simulink library "mmuct_lib"  (R2025a)
settings: Solver=VariableStepAuto  StartTime=0.0  StopTime=10.0  RelTol=1e-3
undefined symbols (not defined in the file): fractalcoef, simstruct, struct2bus
libraries: $bdroot x2, dhaouadi2013_lib x2, mspsensorlib x1
settings Model: Creator=nicolls  LastModifiedBy=MTMTAD006

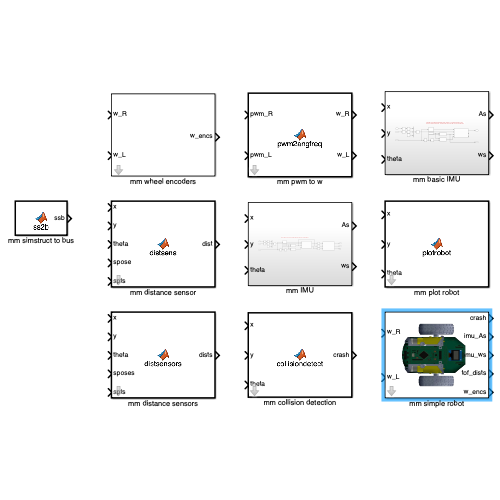
[thumbnail: Simulink's stored preview of the top-level diagram]
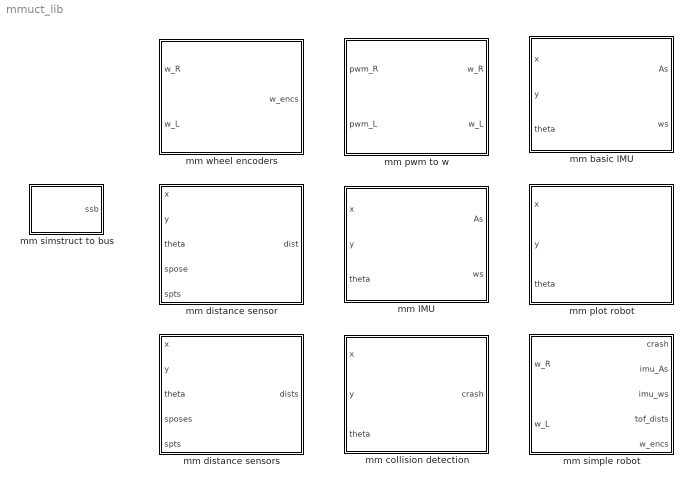
== system mmuct_lib ==
  mm IMU : Subsystem
  mm basic IMU : Subsystem
  mm collision detection : MATLAB Function  InitFcn=struct2bus(simstruct,'ssbus');  TreatAsAtomicUnit=on  mask(MM Collision Detection){simstruct=simstruct}
      mask prompts: simstruct "Simulation structure variable"
      mask help:
      | Detect crash for UCT micromouse at specified pose (x, y, theta) on map.
      |
      | This function uses a simulation structure variable that must include fields "mapim", "mapres", and "robot_rad".
  mm distance sensor : MATLAB Function  InitFcn=struct2bus(simstruct,'ssbus');  TreatAsAtomicUnit=on  mask(MM Distance Sensor){simstruct=simstruct, debug=0}
      mask prompts: simstruct "Simulation structure variable"; debug "Display debugging output"
      mask help:
      | Generate measurement for distance sensor mounted on UCT micro-mouse.  The robot is assumed to be located at pose (x, y, theta) in a map specified by the simulation structure variable.  The sensor is at pose "spose" (x, y, theta) relative to the robot coordinate frame, where the robot kinematic center is at the origin and the forward direction is along the x axis.  The function works by evaluating the map at sensor locations specified by spts, and returns the point corresponding to the closest collision.
      |
      | This function uses a simulation structure variable that must include fields "mapim" and "mapres".
  mm distance sensors : MATLAB Function  InitFcn=struct2bus(simstruct,'ssbus');  TreatAsAtomicUnit=on  mask(MM Distance Sensor){simstruct=simstruct, debug=1}
      mask prompts: simstruct "Simulation structure variable"; debug "Display debugging output"
      mask help:
      | Generate measurement for distance sensor mounted on UCT micro-mouse.  The robot is assumed to be located at pose (x, y, theta) in a map specified by the simulation structure variable.  The sensor is at pose "spose" (x, y, theta) relative to the robot coordinate frame, where the robot kinematic center is at the origin and the forward direction is along the x axis.  The function works by evaluating the map at sensor locations specified by spts, and returns the point corresponding to the closest collision.
      |
      | This function uses a simulation structure variable that must include fields "mapim" and "mapres".
  mm plot robot : MATLAB Function  InitFcn=|  TreatAsAtomicUnit=on  mask(MM Plot Robot){x0=0.1, y0=0.1, theta0=0, simstruct=simstruct}
      | simstruct_var = get_param(gcb,'simstruct'); 
      | existsinbase = evalin('base', ['exist(''' simstruct_var ''',''var'')']); 
      | 
      | ss = [];
      | if existsinbase 
      |   %disp(['initFcn: loading simulation structure ' simstruct_var]); 
      |   ss = evalin('base',simstruct_var); 
      | end
      | struct2bus(ss,'ssbus');  % generate bus definition
      mask prompts: x0 "x0 (m)"; y0 "y0 (m)"; theta0 "theta0 (rad)"; simstruct "Simulation structure variable"
      mask help:
      | Plot UCT micromouse at specified pose (x, y, theta) on map.
      |
      | This function uses a simulation structure variable that must include fields "mapim", "mapres", "robot_img", "robot_imgalpha", and "robot_imgxyd".  It also opens a figure and leaves a handle "UCTMMRobotSimulatorHandle" in the base workspace.
      mask init:
      | FigureName = 'UCT MM Robot Simulator';
      |   FigureTag = 'UCTMMRobotSimulator';
      | 
      |   h = findobj('Name',FigureName);
      |   if ~isempty(h)
      |     close (h); 
      |   end
      | 
      |   % Figure setup
      |   existingFigures = findobj('type','figure','tag',FigureTag);
      |   if ~isempty(existingFigures)
      |     figure(existingFigures(1)); % bring figure to the front
      |     error('There is already an existing figure window for RobotSimulator.');
      |   end
      |   fh = figure('Name',FigureName,'tag',FigureTag);
      |   ax = axes('parent',fh);
      | 
      |   % % Mask parameters
      |   % x0 = str2double(get_param(gcb,'x0'));
      |   % y0 = str2double(get_param(gcb,'y0'));
      |   % theta0 = str2double(get_param(gcb,'theta0'));
      |   % 
      |   % % Determine if simstruct is available
      |   % simstruct = [];
      |   % simstruct_var = get_param(gcb,'simstruct');
      |   % existsinbase = evalin('base', ['exist(''' simstruct_var ''',''var'')']);
      |   % if existsinbase
      |   %   simstruct = evalin('base',simstruct_var);
      |   % end
      | 
      |   % Display map
      |   if isfield(simstruct,'mapim') && isfield(simstruct,'mapres')
      |     map = binaryOccupancyMap(simstruct.mapim,simstruct.mapres);
      |     show(map,'Parent',ax); 
      |   else
      |     axis([-2 2 -2 2]);
      |   end
      | 
      |   % Display robot
      |   if isfield(simstruct,'robot_img') && isfield(simstruct,'robot_imgalpha') && isfield(simstruct,'robot_imgxyd')
      |     % Get robot
      |     robot_img = simstruct.robot_img;
      |     robot_imgalpha = simstruct.robot_imgalpha;
      |     robot_imgxyd = simstruct.robot_imgxyd;
      | 
      |     % Display robot
      |     robot_imgr = imrotate(robot_img,-theta0*180/pi,'crop');
      |     robot_imgalphar = imrotate(robot_imgalpha,-theta0*180/pi,'crop');
      |     hold on;
      |     ih = image(x0+robot_imgxyd,y0+robot_imgxyd,robot_imgr);
      |     set(ih,'AlphaData',robot_imgalphar);
      |     hold off;
      |   else
      |     hold on;  sh = scatter(x0,y0,'ro');  hold off;
      |     llen = 0.25;
      |     hold on;  lh = line([x0; x0+llen*cos(theta0)],[y0;y0+llen*sin(theta0)]);  hold off;
      |     ih = [sh lh];
      |   end
      | 
      |   % Store handles 
      |   set(fh,'UserData',ih);
      |   assignin('base','UCTMMRobotSimulatorHandle',fh);
  mm pwm to w : MATLAB Function  TreatAsAtomicUnit=on  mask{deadb=30, maxw=2*pi}
      mask prompts: deadb "Dead band (%)"; maxw "Max. angular velocity (rad/s)"
  mm simple robot : Subsystem  mask{simstruct=simstruct, x0=0.1, y0=0.1, theta0=0}
      mask prompts: simstruct "Simulation structure variable"; x0 "x0 (m)"; y0 "y0 (m)"; theta0 "theta0 (rad)"
      mask DialogControl Container3 Prompt: Initial pose
      mask Display: image('uctmm_image.png');
  mm simstruct to bus : MATLAB Function  InitFcn=struct2bus(simstruct,'ssbus')  TreatAsAtomicUnit=on
  mm wheel encoders : Subsystem  mask{ticsperrev=12}
      mask prompts: ticsperrev "Tics/rev"

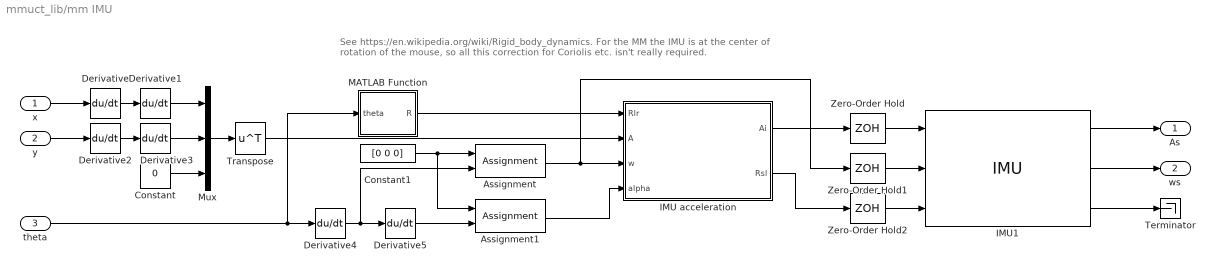
== system mmuct_lib/mm IMU ==
  note: See https://en.wikipedia.org/wiki/Rigid_body_dynamics. For the MM the IMU is at the center of rotation of the mouse, so all this correction for Coriolis etc. isn't really required.
  x : Inport
  y : Inport  Port=2
  theta : Inport  Port=3
  Assignment : Assignment  DiagnosticForDimensions=Warning  IndexOptions=Index vector (dialog)  Indices=3  OutputSizes=1
  Assignment1 : Assignment  DiagnosticForDimensions=Warning  IndexOptions=Index vector (dialog)  Indices=3  OutputSizes=1
  Constant : Constant  Value=0
  Constant1 : Constant  Value=[0 0 0]  VectorParams1D=off
  Derivative{,1..5} (6 alike) : Derivative
  IMU acceleration : MATLAB Function  TreatAsAtomicUnit=on
  IMU1 : mspsensorlib/IMU  DispRefFrame=ENU  TemperaturePort=off  Temperature=25  MagneticFieldPort=off  MagneticFieldNED=[ 27.5550, -2.4169, -16.0849 ]  MagneticFieldENU=[ -2.4169, 27.5550, 16.0849 ]  SeedDouble=67  SimulateUsing=Interpreted execution  AccelParamsMeasurementRange=Inf  AccelParamsResolution=0  AccelParamsConstantBias=[ 0, 0, 0 ]  AccelParamsAxesMisalignment=[ 100, 0, 0; 0, 100, 0; 0, 0, 100 ]  AccelParamsNoiseDensity=[ 0, 0, 0 ]  AccelParamsBiasInstability=[ 0, 0, 0 ]  AccelParamsBiasInstabilityNumerator=fractalcoef().Numerator  AccelParamsBiasInstabilityDenominator=fractalcoef().Denominator  AccelParamsRandomWalk=[ 0, 0, 0 ]  AccelParamsNoiseType=double-sided  AccelParamsTemperatureBias=[ 0, 0, 0 ]  AccelParamsTemperatureScaleFactor=[ 0, 0, 0 ]  GyroParamsMeasurementRange=Inf  GyroParamsResolution=0  GyroParamsConstantBias=[ 0, 0, 0 ]  GyroParamsAxesMisalignment=[ 100, 0, 0; 0, 100, 0; 0, 0, 100 ]  GyroParamsAccelerationBias=[ 0, 0, 0 ]  GyroParamsNoiseDensity=[ 0, 0, 0 ]  GyroParamsBiasInstability=[ 0, 0, 0 ]  GyroParamsBiasInstabilityNumerator=fractalcoef().Numerator  GyroParamsBiasInstabilityDenominator=fractalcoef().Denominator  GyroParamsRandomWalk=[ 0, 0, 0 ]  GyroParamsNoiseType=double-sided  GyroParamsTemperatureBias=[ 0, 0, 0 ]  GyroParamsTemperatureScaleFactor=[ 0, 0, 0 ]  MagParamsMeasurementRange=Inf  MagParamsResolution=0  MagParamsConstantBias=[ 0, 0, 0 ]  MagParamsAxesMisalignment=[ 100, 0, 0; 0, 100, 0; 0, 0, 100 ]  MagParamsNoiseDensity=[ 0, 0, 0 ]  MagParamsBiasInstability=[ 0, 0, 0 ]  MagParamsBiasInstabilityNumerator=fractalcoef().Numerator  MagParamsBiasInstabilityDenominator=fractalcoef().Denominator  MagParamsRandomWalk=[ 0, 0, 0 ]  MagParamsNoiseType=double-sided  MagParamsTemperatureBias=[ 0, 0, 0 ]  MagParamsTemperatureScaleFactor=[ 0, 0, 0 ]
  MATLAB Function : MATLAB Function  TreatAsAtomicUnit=on
  Mux : Mux  Inputs=3
  Terminator : Terminator
  Transpose : Math  Operator=transpose
  Zero-Order Hold : ZeroOrderHold  SampleTime=0.02
  Zero-Order Hold1 : ZeroOrderHold  SampleTime=0.02
  Zero-Order Hold2 : ZeroOrderHold  SampleTime=0.02
  As : Outport
  ws : Outport  Port=2
  wires:
  IMU acceleration/2(Rsl) -> Zero-Order Hold2/1
  Mux/1 -> Transpose/1
  IMU acceleration/1(Ai) -> Zero-Order Hold/1
  Zero-Order Hold/1 -> IMU1/1
  Zero-Order Hold1/1 -> IMU1/2
  IMU1/1 -> As/1
  Zero-Order Hold2/1 -> IMU1/3
  x/1 -> Derivative/1
  Derivative/1 -> Derivative1/1
  Derivative2/1 -> Derivative3/1
  y/1 -> Derivative2/1
  Derivative1/1 -> Mux/1
  Derivative3/1 -> Mux/2
  Constant/1 -> Mux/3
  IMU1/2 -> ws/1
  theta/1 -> MATLAB Function/1(theta), Derivative4/1
  MATLAB Function/1(R) -> IMU acceleration/1(Rlr)
  Constant1/1 -> Assignment1/1, Assignment/1
  Derivative4/1 -> Assignment/2, Derivative5/1
  Assignment/1 -> Zero-Order Hold1/1, IMU acceleration/3(w)
  Derivative5/1 -> Assignment1/2
  Assignment1/1 -> IMU acceleration/4(alpha)
  Transpose/1 -> IMU acceleration/2(A)
  IMU1/3 -> Terminator/1

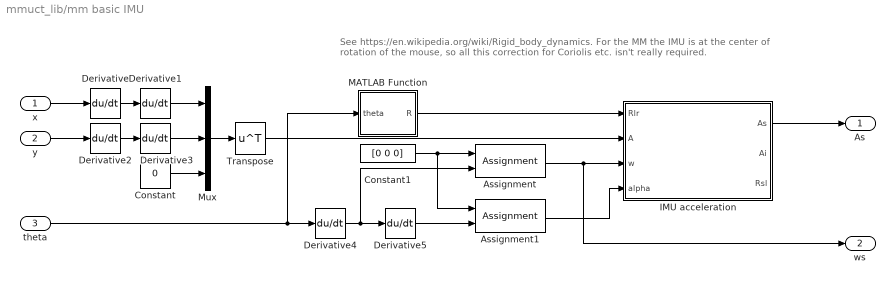
== system mmuct_lib/mm basic IMU ==
  note: See https://en.wikipedia.org/wiki/Rigid_body_dynamics. For the MM the IMU is at the center of rotation of the mouse, so all this correction for Coriolis etc. isn't really required.
  x : Inport
  y : Inport  Port=2
  theta : Inport  Port=3
  Assignment : Assignment  DiagnosticForDimensions=Warning  IndexOptions=Index vector (dialog)  Indices=3  OutputSizes=1
  Assignment1 : Assignment  DiagnosticForDimensions=Warning  IndexOptions=Index vector (dialog)  Indices=3  OutputSizes=1
  Constant : Constant  Value=0
  Constant1 : Constant  Value=[0 0 0]  VectorParams1D=off
  Derivative{,1..5} (6 alike) : Derivative
  IMU acceleration : MATLAB Function  TreatAsAtomicUnit=on
  MATLAB Function : MATLAB Function  TreatAsAtomicUnit=on
  Mux : Mux  Inputs=3
  Transpose : Math  Operator=transpose
  As : Outport
  ws : Outport  Port=2
  wires:
  Assignment1/1 -> IMU acceleration/4(alpha)
  Derivative5/1 -> Assignment1/2
  Assignment/1 -> ws/1, IMU acceleration/3(w)
  Derivative4/1 -> Derivative5/1, Assignment/2
  Constant1/1 -> Assignment/1, Assignment1/1
  MATLAB Function/1(R) -> IMU acceleration/1(Rlr)
  theta/1 -> Derivative4/1, MATLAB Function/1(theta)
  Constant/1 -> Mux/3
  Derivative3/1 -> Mux/2
  Derivative1/1 -> Mux/1
  y/1 -> Derivative2/1
  Derivative2/1 -> Derivative3/1
  Derivative/1 -> Derivative1/1
  x/1 -> Derivative/1
  Mux/1 -> Transpose/1
  Transpose/1 -> IMU acceleration/2(A)
  IMU acceleration/1(As) -> As/1

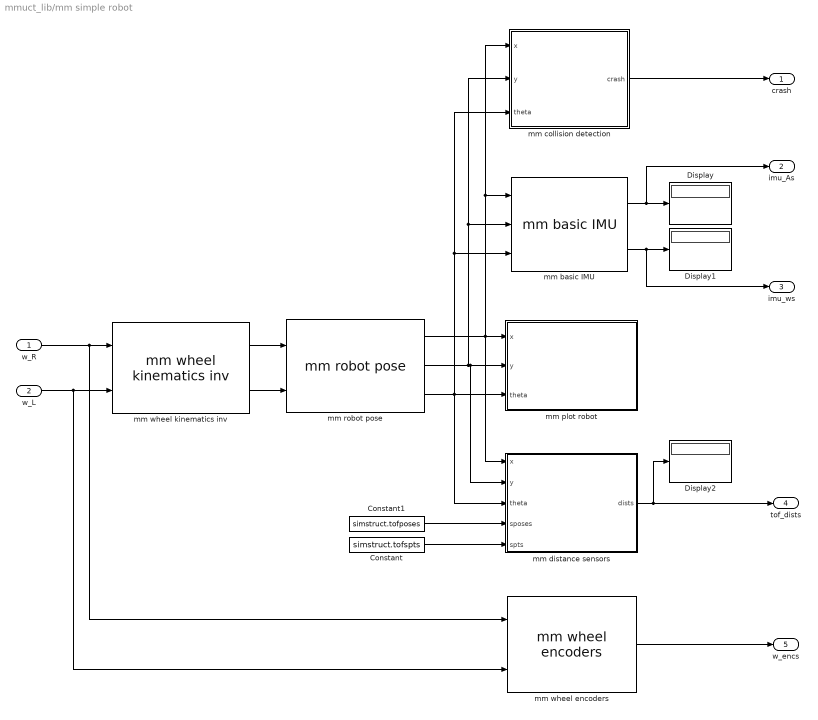
== system mmuct_lib/mm simple robot ==
  w_R : Inport
  w_L : Inport  Port=2
  Constant : Constant  Value=simstruct.tofspts
  Constant1 : Constant  Value=simstruct.tofposes
  Display : Display
  Display1 : Display
  Display2 : Display
  mm basic IMU : $bdroot/mm basic IMU  SystemSampleTime=-1  VariantActivationTime=update diagram  EmptyChoice=off  PassThrough=off  PassThroughVariantControl=(default)  EmptyChoiceVariantControl=(default)  AllowFlexibleInterface=on  Latency=0  AutoFrameSizeCalculation=off
  mm collision detection : MATLAB Function  InitFcn=struct2bus(simstruct,'ssbus');  TreatAsAtomicUnit=on  mask(MM Collision Detection){simstruct=simstruct}
      mask prompts: simstruct "Simulation structure variable"
      mask help:
      | Detect crash for UCT micromouse at specified pose (x, y, theta) on map.
      |
      | This function uses a simulation structure variable that must include fields "mapim", "mapres", and "robot_rad".
  mm distance sensors : MATLAB Function  InitFcn=struct2bus(simstruct,'ssbus');  TreatAsAtomicUnit=on  mask(MM Distance Sensor){simstruct=simstruct, debug=0}
      mask prompts: simstruct "Simulation structure variable"; debug "Display debugging output"
      mask help:
      | Generate measurement for distance sensor mounted on UCT micro-mouse.  The robot is assumed to be located at pose (x, y, theta) in a map specified by the simulation structure variable.  The sensor is at pose "spose" (x, y, theta) relative to the robot coordinate frame, where the robot kinematic center is at the origin and the forward direction is along the x axis.  The function works by evaluating the map at sensor locations specified by spts, and returns the point corresponding to the closest collision.
      |
      | This function uses a simulation structure variable that must include fields "mapim" and "mapres".
  mm plot robot : MATLAB Function  InitFcn=|  TreatAsAtomicUnit=on  mask(MM Plot Robot){x0=x0, y0=y0, theta0=theta0, simstruct=simstruct}
      | simstruct_var = get_param(gcb,'simstruct'); 
      | existsinbase = evalin('base', ['exist(''' simstruct_var ''',''var'')']); 
      | 
      | ss = [];
      | if existsinbase 
      |   %disp(['initFcn: loading simulation structure ' simstruct_var]); 
      |   ss = evalin('base',simstruct_var); 
      | end
      | struct2bus(ss,'ssbus');  % generate bus definition
      mask prompts: x0 "x0 (m)"; y0 "y0 (m)"; theta0 "theta0 (rad)"; simstruct "Simulation structure variable"
      mask help:
      | Plot UCT micromouse at specified pose (x, y, theta) on map.
      |
      | This function uses a simulation structure variable that must include fields "mapim", "mapres", "robot_img", "robot_imgalpha", and "robot_imgxyd".  It also opens a figure and leaves a handle "UCTMMRobotSimulatorHandle" in the base workspace.
      mask init: same as mmuct_lib/mm plot robot
  mm robot pose : dhaouadi2013_lib/mm robot pose  x0=x0  y0=y0  theta0=0
  mm wheel encoders : $bdroot/mm wheel encoders  ticsperrev=8
  mm wheel kinematics inv : dhaouadi2013_lib/mm wheel kinematics inv  L=simstruct.L  R=simstruct.R
  crash : Outport
  imu_As : Outport  Port=2
  imu_ws : Outport  Port=3
  tof_dists : Outport  Port=4
  w_encs : Outport  Port=5
  wires:
  mm wheel encoders/1 -> w_encs/1
  mm distance sensors/1(dists) -> tof_dists/1, Display2/1
  Constant/1 -> mm distance sensors/5(spts)
  Constant1/1 -> mm distance sensors/4(sposes)
  mm wheel kinematics inv/2 -> mm robot pose/2
  mm robot pose/2 -> mm plot robot/2(y), mm distance sensors/2(y), mm collision detection/2(y), mm basic IMU/2
  mm basic IMU/2 -> imu_ws/1, Display1/1
  mm basic IMU/1 -> Display/1, imu_As/1
  mm wheel kinematics inv/1 -> mm robot pose/1
  mm robot pose/1 -> mm plot robot/1(x), mm basic IMU/1, mm collision detection/1(x), mm distance sensors/1(x)
  mm robot pose/3 -> mm plot robot/3(theta), mm collision detection/3(theta), mm basic IMU/3, mm distance sensors/3(theta)
  mm collision detection/1(crash) -> crash/1
  w_L/1 -> mm wheel kinematics inv/2, mm wheel encoders/2
  w_R/1 -> mm wheel kinematics inv/1, mm wheel encoders/1

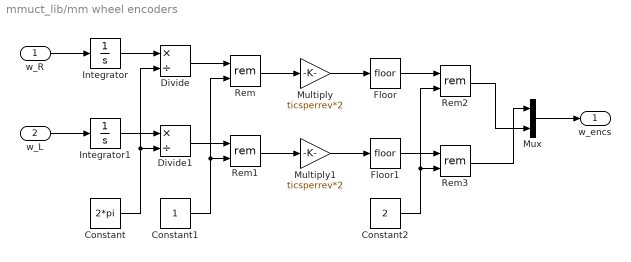
== system mmuct_lib/mm wheel encoders ==
  w_R : Inport
  w_L : Inport  Port=2
  Constant : Constant  Value=2*pi
  Constant1 : Constant
  Constant2 : Constant  Value=2
  Divide : Product  Inputs=*/
  Divide1 : Product  Inputs=*/
  Floor : Rounding
  Floor1 : Rounding
  Integrator : Integrator
  Integrator1 : Integrator
  Multiply : Gain  Gain=ticsperrev*2
  Multiply1 : Gain  Gain=ticsperrev*2
  Mux : Mux  Inputs=2
  Rem{,1..3} (4 alike) : Math  Operator=rem
  w_encs : Outport
  wires:
  Mux/1 -> w_encs/1
  Rem3/1 -> Mux/1
  Rem2/1 -> Mux/2
  Constant2/1 -> Rem2/2, Rem3/2
  Floor/1 -> Rem2/1
  Floor1/1 -> Rem3/1
  Multiply1/1 -> Floor1/1
  Multiply/1 -> Floor/1
  Rem/1 -> Multiply/1
  Rem1/1 -> Multiply1/1
  Constant1/1 -> Rem/2, Rem1/2
  Divide1/1 -> Rem1/1
  Divide/1 -> Rem/1
  Constant/1 -> Divide/2, Divide1/2
  Integrator1/1 -> Divide1/1
  Integrator/1 -> Divide/1
  w_L/1 -> Integrator1/1
  w_R/1 -> Integrator/1

== matlab function mmuct_lib/mm distance sensors ==
  data: x input; y input; theta input; dists output; sposes input; spts input; simstruct parameter; debug parameter
function dists = distsensors(x,y,theta,sposes,spts,simstruct,debug)
%DISTSENS  Simulate output of time-of-flight distance sensor
%   dists = distsens(x,y,theta,sposes,spts,simstruct,debug) takes a
%   robot pose in the world (x, y, theta), a sensor pose in the robot frame
%   (spos), and a set of sensor points to be checked in the sensor frame,
%   and finds the distance from the sensor to the nearest sensor point that
%   collides with an occupied cell on a map. 
%
%   Parameters:
%     x, y, theta - robot pose in world
%     sposes - sensor poses in robot frame (one row [x y theta] for each
%              sensor).  It is assumed that the robot is centered at the
%              origin and is pointing forwards along the x axis 
%     spts - set of points in sensor frame for which to detect collisions.
%            Must be increasing and should be spaced closely enough for
%            collisions to be detected
%     simstruct - simulation structure assumed to have field mapim for map
%                 occupancy image (zero for cell unoccupied), at a map
%                 resolution mapres (pixels per meter)
%     debug - display interesting plot
%
%   Fred Nicolls, July 2025

coder.extrinsic('get_param','set_param');

rpose = [x y theta]';
if numel(rpose)~=3, error('Invalid dimension'); end
if size(sposes,2)~=3, error('Invalid dimension'); end
if any(diff(spts)<0), error('Sensor points must be increasing'); end
if nargin<7, debug=0; end
numsens = size(sposes,1);

% Transpose inputs if required
if size(rpose,1)==1, rpose = rpose'; end
if size(spts,1)==1, sptsr = spts;  else sptsr = spts'; end

% Points in sensor frame lying on x-axis
xs = [sptsr; zeros(size(sptsr))];

% Robot to world coordinate transformation
thetar = rpose(3);  xyr = rpose(1:2);
Rwr = [cos(thetar) -sin(thetar) xyr(1); sin(thetar) cos(thetar) xyr(2); 0 0 1];

% Collect sensor information in cells
Rrsc = cell(numsens,1);
xwsc = cell(numsens,1);
xwc = cell(numsens,1);

% For each sensor
for i=1:numsens

  % Sensor to robot coordinate transformation
  thetas = sposes(i,3);  xys = sposes(i,1:2);
  Rrs = [cos(thetas) -sin(thetas) xys(1); sin(thetas) cos(thetas) xys(2); 0 0 1];

  % Get sensor point in world
  xwsh = Rwr*Rrs*[0; 0; 1];
  xws = xwsh(1:2)/xwsh(3);

  % Get sensor sample points in world
  xsh = [xs; ones(1,size(xs,2))];
  xwh = Rwr*Rrs*xsh;
  xw = xwh(1:2,:)./repmat(xwh(3,:),2,1);

  % Store
  Rrsc{i} = Rrs;  xwsc{i} = xws;  xwc{i} = xw;

end

% Map image and resolution
mapim = simstruct.mapimfud;
mapres = simstruct.mapres;

% Get sensor sample points in map image
xwa = cat(2,xwc{:});  % all points at once
xia = round(mapres*xwa) + 1;
xira = xia(1,:);  yira = xia(2,:);

% Valid points in map domain
ii = xira>=1 & xira<=size(mapim,2) & yira>=1 & yira<=size(mapim,1);

% Get values for each point
mpv = zeros(size(ii));  % value of zero for points outside map
mpv(ii) = mapim(sub2ind(size(mapim),yira(ii),xira(ii)));

% Split results for each sensor
mpvm = reshape(mpv,[],numsens)';
mpvc = cell(numsens,1);
for i=1:numsens, mpvc{i} = mpvm(i,:); end

% Get collision points and distances
dists = zeros(numsens,1);
xwcollc = cell(numsens,1);
for i=1:numsens
  xw = xwc{i};  xws = xwsc{i};  mpv = mpvc{i};

  % Find first nonzero sample 
  dist = NaN;  xwcoll = [NaN; NaN];
  k = find(mpv,1,'first');
  if ~isempty(k) && k(1)~=0
    xwcoll = xw(:,k(1));  % collision point in world
    dist = sqrt(sum((xwcoll - xws).^2));
  end

  dists(i) = dist;  xwcollc{i} = xwcoll;
end

% Plot to debug
if debug
  % Draw map
  fh = figure;  
  ih = imagesc((1:size(mapim,2)-1)/mapres,(1:size(mapim,1)-1)/mapres,mapim==0);
  colormap(gray);  axis equal;  axis tight;  axis xy;
  title('Distsensors debug');

  % Draw robot
  rpp = [0 0.2; 0 0];
  rpwh = Rwr*[rpp; ones(1,size(rpp,2))];
  rpw = rpwh(1:2,:)./repmat(rpwh(3,:),2,1);
  hold on;  
  sh = scatter(rpw(1,1),rpw(2,1),'ro');  
  lh = line(rpw(1,:),rpw(2,:));  
  hold off;
  
  % Draw sensor points
  for i=1:numsens
    xws = xwsc{i};
    figure(fh);
    hold on;  sh = scatter(xws(1,:),xws(2,:),'bo');  hold off;
  end

  % Draw sensor lines
  for i=1:numsens
    xw = xwc{i};
    figure(fh);
    hold on;  sh = scatter(xw(1,:),xw(2,:),'b.');  hold off;
  end

  % Draw collision points
  for i=1:numsens
    xwcoll = xwcollc{i};
    hold on;  sh = scatter(xwcoll(1),xwcoll(2),'gx');  hold off;
    set(sh,'SizeData',100,'LineWidth',2);
  end

  % Terminate simulation to prevent too many figure windows
  %modelName = get_param(bdroot, 'Name');
  %set_param(modelName,'SimulationCommand','stop');
  error('Terminating simulation to prevent too many figures');
end

== matlab function mmuct_lib/mm simple robot/mm plot robot ==
  data: x input; y input; theta input; simstruct parameter Bus: ssbus
function plotrobot(x,y,theta,simstruct)
coder.extrinsic('imread', 'image', 'set', 'drawnow', 'evalin', 'plot', 'keyboard');
%persistent plotHandle robot_img robot_imgalpha robot_imgres robot_imgxyd;

fh = evalin('base','UCTMMRobotSimulatorHandle');
ih = get(fh,'UserData');

if isfield(simstruct,'robot_img') && isfield(simstruct,'robot_imgalpha') && isfield(simstruct,'robot_imgxyd')
  robot_img = simstruct.robot_img;
  robot_imgalpha = simstruct.robot_imgalpha;
  robot_imgxyd = simstruct.robot_imgxyd;

  % Display rotated robot image
  robot_imgr = imrotate(robot_img,-theta*180/pi,'crop');
  robot_imgalphar = imrotate(robot_imgalpha,-theta*180/pi,'crop');
  set(ih,'CData',robot_imgr,'AlphaData',robot_imgalphar,'XData',x+robot_imgxyd,'YData',y+robot_imgxyd);
else
  sh = ih(1);  lh = ih(2);
  set(sh,'XData',x,'YData',y);
  llen = 0.25;
  set(lh,'XData',[x; x+llen*cos(theta)],'YData',[y;y+llen*sin(theta)]);
end
drawnow('limitrate', 'nocallbacks');

== matlab function mmuct_lib/mm simple robot/mm collision detection ==
  data: x input; crash output; y input; theta input; simstruct parameter Bus: ssbus
function crash = collisiondetect(x,y,theta,simstruct)
coder.extrinsic('imread', 'image', 'set', 'drawnow', 'evalin', 'plot');

mapdt = simstruct.mapdt;
mapres = simstruct.mapres;
robot_rad = simstruct.robot_rad;

crash = 0;

% Always crashed if out of map
xi = x*mapres + 1;  yi = round(y*mapres) + 1;  % world to image
if yi<1 || yi>size(mapdt,1) || xi<1 || xi>size(mapdt,2)
  crash = 1;
  return;
end

% Crash if too close to wall
dist = mapdt(sub2ind(size(mapdt),yi,xi));
if dist<robot_rad
  crash = 1;
end

== matlab function mmuct_lib/mm basic IMU/MATLAB Function ==
  data: theta input; R output
function R = theta2R(theta)

R = axang2rotm([0 0 1 theta]);

== matlab function mmuct_lib/mm plot robot ==
  data: x input; y input; theta input; simstruct parameter Bus: ssbus
function plotrobot(x,y,theta,simstruct)
coder.extrinsic('imread', 'image', 'set', 'drawnow', 'evalin', 'plot', 'keyboard');
%persistent plotHandle robot_img robot_imgalpha robot_imgres robot_imgxyd;

fh = evalin('base','UCTMMRobotSimulatorHandle');
ih = get(fh,'UserData');

if isfield(simstruct,'robot_img') && isfield(simstruct,'robot_imgalpha') && isfield(simstruct,'robot_imgxyd')
  robot_img = simstruct.robot_img;
  robot_imgalpha = simstruct.robot_imgalpha;
  robot_imgxyd = simstruct.robot_imgxyd;

  % Display rotated robot image
  robot_imgr = imrotate(robot_img,-theta*180/pi,'crop');
  robot_imgalphar = imrotate(robot_imgalpha,-theta*180/pi,'crop');
  set(ih,'CData',robot_imgr,'AlphaData',robot_imgalphar,'XData',x+robot_imgxyd,'YData',y+robot_imgxyd);
else
  sh = ih(1);  lh = ih(2);
  set(sh,'XData',x,'YData',y);
  llen = 0.25;
  set(lh,'XData',[x; x+llen*cos(theta)],'YData',[y;y+llen*sin(theta)]);
end
drawnow('limitrate', 'nocallbacks');

== matlab function mmuct_lib/mm distance sensor ==
  data: x input; y input; theta input; dist output; spose input; spts input; simstruct parameter; debug parameter
function dist = distsens(x,y,theta,spose,spts,simstruct,debug)
%DISTSENS  Simulate output of time-of-flight distance sensor
%   dist = distsens(x,y,theta,spose,spts,simstruct,debug) takes a
%   robot pose in the world (x, y, theta), a sensor pose in the robot frame
%   (spos), and a set of sensor points to be checked in the sensor frame,
%   and finds the distance from the sensor to the nearest sensor point that
%   collides with an occupied cell on a map. 
%
%   Parameters:
%     x, y, theta - robot pose in world
%     spose - sensor pose in robot frame ([x y theta]).  It is assumed that
%             the robot is centered at the origin and is pointing forwards
%             along the x axis
%     spts - set of points in sensor frame for which to detect collisions.
%            Must be increasing and should be spaced closely enough for
%            collisions to be detected
%     simstruct - simulation structure assumed to have field mapim for map
%                 occupancy image (zero for cell unoccupied), at a map
%                 resolution mapres (pixels per meter)
%     debug - display interesting plot
%
%   Fred Nicolls, July 2025

coder.extrinsic('get_param','set_param');

rpose = [x y theta]';
if numel(rpose)~=3, error('Invalid dimension'); end
if numel(spose)~=3, error('Invalid dimension'); end
if any(diff(spts)<0), error('Sensor points must be increasing'); end
if nargin<7, debug=0; end

% Transpose inputs if required
if size(rpose,1)==1, rpose = rpose'; end
if size(spose,1)==1, spose = spose'; end
if size(spts,1)==1, sptsr = spts;  else sptsr = spts'; end

% Points in sensor frame lying on x-axis
xs = [sptsr; zeros(size(sptsr))];

% Robot to world coordinate transformation
thetar = rpose(3);  xyr = rpose(1:2);
Rwr = [cos(thetar) -sin(thetar) xyr(1); sin(thetar) cos(thetar) xyr(2); 0 0 1];

% Sensor to robot coordinate transformation
thetas = spose(3);  xys = spose(1:2);
Rrs = [cos(thetas) -sin(thetas) xys(1); sin(thetas) cos(thetas) xys(2); 0 0 1];

% Get sensor point in world
xwsh = Rwr*Rrs*[0; 0; 1];
xws = xwsh(1:2)/xwsh(3);

% Get sensor sample points in world
xsh = [xs; ones(1,size(xs,2))];
xwh = Rwr*Rrs*xsh;
xw = xwh(1:2,:)./repmat(xwh(3,:),2,1);

% Map image and resolution
mapim = simstruct.mapimfud;
mapres = simstruct.mapres;

% Get sensor sample points in map image
xi = round(mapres*xw) + 1;
xir = xi(1,:);  yir = xi(2,:);

% Valid points in map domain
ii = xir>=1 & xir<=size(mapim,2) & yir>=1 & yir<=size(mapim,1);

% Get values for each point
mpv = zeros(size(ii));  % value of zero for points outside map
mpv(ii) = mapim(sub2ind(size(mapim),yir(ii),xir(ii)));

% Find first nonzero sample 
dist = NaN;  xwc = [NaN; NaN];
k = find(mpv,1,'first');
if ~isempty(k) && k(1)~=0
  xwc = xw(:,k(1));  % collision point in world
  dist = sqrt(sum((xwc - xws).^2));
end

% Plot to debug
if debug
  % Draw map
  fh = figure;  
  ih = imagesc((1:size(mapim,2)-1)/mapres,(1:size(mapim,1)-1)/mapres,mapim==0);
  colormap(gray);  axis equal;  axis tight;  axis xy;

  % Draw robot
  rpp = [0 0.2; 0 0];
  rpwh = Rwr*[rpp; ones(1,size(rpp,2))];
  rpw = rpwh(1:2,:)./repmat(rpwh(3,:),2,1);
  hold on;  
  sh = scatter(rpw(1,1),rpw(2,1),'ro');  
  lh = line(rpw(1,:),rpw(2,:));  
  hold off;
  
  % Draw sensor, sensor line, and collision point
  hold on;  sh = scatter(xws(1,:),xws(2,:),'bo');  hold off;
  hold on;  sh = scatter(xw(1,:),xw(2,:),'b.');  hold off;
  hold on;  sh = scatter(xwc(1),xwc(2),'gx');  hold off;
  set(sh,'SizeData',100,'LineWidth',2);

  % Terminate simulation to prevent too many figure windows
  %modelName = get_param(bdroot, 'Name');
  %set_param(modelName,'SimulationCommand','stop');
  error('Terminating simulation to prevent too many figures');
end

== matlab function mmuct_lib/mm collision detection ==
  data: x input; crash output; y input; theta input; simstruct parameter Bus: ssbus
function crash = collisiondetect(x,y,theta,simstruct)
coder.extrinsic('imread', 'image', 'set', 'drawnow', 'evalin', 'plot');

mapdt = simstruct.mapdt;
mapres = simstruct.mapres;
robot_rad = simstruct.robot_rad;

crash = 0;

% Always crashed if out of map
xi = x*mapres + 1;  yi = round(y*mapres) + 1;  % world to image
if yi<1 || yi>size(mapdt,1) || xi<1 || xi>size(mapdt,2)
  crash = 1;
  return;
end

% Crash if too close to wall
dist = mapdt(sub2ind(size(mapdt),yi,xi));
if dist<robot_rad
  crash = 1;
end

== matlab function mmuct_lib/mm IMU/IMU acceleration ==
  data: Ai output; Rsl output; Rlr input; A input; w input; alpha input; simstruct parameter
function [Ai,Rsl]  = getimuaccel(Rlr,A,w,alpha,simstruct)
%GETIMUACCEL  Get linear acceleration of IMU in local frame
%  [Ai,Rls]  = getimuaccel(Rlr,A,w,alpha,simstruct) calculates the linear
%  acceleration at the origin of an IMU sensor frame fixed to a robot.  The
%  robot frame is oriented by Rlr with respect to the local frane and is
%  moving according to (A,w,alpha) = (linear acceleration,angular
%  velocity,anglular acceleration). 
%
%  The function returns the linear acceleration As and the orientation Rsl
%  of the local frame in the sensor frame.  These two outputs are useful
%  for setting up the standard Simulink IMU block.

% Checks
if size(A,1)~=1 || size(A,2)~=3, error('Input A must be 1x3'); end
if size(w,1)~=1 || size(w,2)~=3, error('Input w must be 1x3'); end
if size(alpha,1)~=1 || size(alpha,2)~=3, error('Input alpha must be 1x3'); end

% Get sensor location vector (r_i-R) in local frame
si = Rlr*simstruct.timu;

% Kinematic equation (https://en.wikipedia.org/wiki/Rigid_body_dynamics,
% taking R as origin of robot frame).  This find the linear acceleration of
% the IMU in the local (inertial) navigation frame 
Ai = cross(alpha,si) + cross(w,cross(w,si)) + A;

% Get sensor orientation in local frame
Rrs = simstruct.Rimu;
Rls = Rlr*Rrs;
Rsl = inv(Rls);

% Generate measurements in sensor frame
Ait = Ai;  Ait(3) = Ait(3) + 9.81;  % add gravity
As = (inv(Rls)*Ait')';  
ws = (inv(Rls)*w')';

== matlab function mmuct_lib/mm IMU/MATLAB Function ==
  data: theta input; R output
function R = theta2R(theta)

R = axang2rotm([0 0 1 theta]);

== matlab function mmuct_lib/mm simstruct to bus ==
  data: ssb output Bus: ssbus
function ssb = ss2b()
coder.extrinsic('evalin');

ssb = evalin('base','simstruct');

== matlab function mmuct_lib/mm simple robot/mm distance sensors ==
  data: x input; y input; theta input; dists output; sposes input; spts input; simstruct parameter; debug parameter
function dists = distsensors(x,y,theta,sposes,spts,simstruct,debug)
%DISTSENS  Simulate output of time-of-flight distance sensor
%   dists = distsens(x,y,theta,sposes,spts,simstruct,debug) takes a
%   robot pose in the world (x, y, theta), a sensor pose in the robot frame
%   (spos), and a set of sensor points to be checked in the sensor frame,
%   and finds the distance from the sensor to the nearest sensor point that
%   collides with an occupied cell on a map. 
%
%   Parameters:
%     x, y, theta - robot pose in world
%     sposes - sensor poses in robot frame (one row [x y theta] for each
%              sensor).  It is assumed that the robot is centered at the
%              origin and is pointing forwards along the x axis 
%     spts - set of points in sensor frame for which to detect collisions.
%            Must be increasing and should be spaced closely enough for
%            collisions to be detected
%     simstruct - simulation structure assumed to have field mapim for map
%                 occupancy image (zero for cell unoccupied), at a map
%                 resolution mapres (pixels per meter)
%     debug - display interesting plot
%
%   Fred Nicolls, July 2025

coder.extrinsic('get_param','set_param');

rpose = [x y theta]';
if numel(rpose)~=3, error('Invalid dimension'); end
if size(sposes,2)~=3, error('Invalid dimension'); end
if any(diff(spts)<0), error('Sensor points must be increasing'); end
if nargin<7, debug=0; end
numsens = size(sposes,1);

% Transpose inputs if required
if size(rpose,1)==1, rpose = rpose'; end
if size(spts,1)==1, sptsr = spts;  else sptsr = spts'; end

% Points in sensor frame lying on x-axis
xs = [sptsr; zeros(size(sptsr))];

% Robot to world coordinate transformation
thetar = rpose(3);  xyr = rpose(1:2);
Rwr = [cos(thetar) -sin(thetar) xyr(1); sin(thetar) cos(thetar) xyr(2); 0 0 1];

% Collect sensor information in cells
Rrsc = cell(numsens,1);
xwsc = cell(numsens,1);
xwc = cell(numsens,1);

% For each sensor
for i=1:numsens

  % Sensor to robot coordinate transformation
  thetas = sposes(i,3);  xys = sposes(i,1:2);
  Rrs = [cos(thetas) -sin(thetas) xys(1); sin(thetas) cos(thetas) xys(2); 0 0 1];

  % Get sensor point in world
  xwsh = Rwr*Rrs*[0; 0; 1];
  xws = xwsh(1:2)/xwsh(3);

  % Get sensor sample points in world
  xsh = [xs; ones(1,size(xs,2))];
  xwh = Rwr*Rrs*xsh;
  xw = xwh(1:2,:)./repmat(xwh(3,:),2,1);

  % Store
  Rrsc{i} = Rrs;  xwsc{i} = xws;  xwc{i} = xw;

end

% Map image and resolution
mapim = simstruct.mapimfud;
mapres = simstruct.mapres;

% Get sensor sample points in map image
xwa = cat(2,xwc{:});  % all points at once
xia = round(mapres*xwa) + 1;
xira = xia(1,:);  yira = xia(2,:);

% Valid points in map domain
ii = xira>=1 & xira<=size(mapim,2) & yira>=1 & yira<=size(mapim,1);

% Get values for each point
mpv = zeros(size(ii));  % value of zero for points outside map
mpv(ii) = mapim(sub2ind(size(mapim),yira(ii),xira(ii)));

% Split results for each sensor
mpvm = reshape(mpv,[],numsens)';
mpvc = cell(numsens,1);
for i=1:numsens, mpvc{i} = mpvm(i,:); end

% Get collision points and distances
dists = zeros(numsens,1);
xwcollc = cell(numsens,1);
for i=1:numsens
  xw = xwc{i};  xws = xwsc{i};  mpv = mpvc{i};

  % Find first nonzero sample 
  dist = NaN;  xwcoll = [NaN; NaN];
  k = find(mpv,1,'first');
  if ~isempty(k) && k(1)~=0
    xwcoll = xw(:,k(1));  % collision point in world
    dist = sqrt(sum((xwcoll - xws).^2));
  end

  dists(i) = dist;  xwcollc{i} = xwcoll;
end

% Plot to debug
if debug
  % Draw map
  fh = figure;  
  ih = imagesc((1:size(mapim,2)-1)/mapres,(1:size(mapim,1)-1)/mapres,mapim==0);
  colormap(gray);  axis equal;  axis tight;  axis xy;
  title('Distsensors debug');

  % Draw robot
  rpp = [0 0.2; 0 0];
  rpwh = Rwr*[rpp; ones(1,size(rpp,2))];
  rpw = rpwh(1:2,:)./repmat(rpwh(3,:),2,1);
  hold on;  
  sh = scatter(rpw(1,1),rpw(2,1),'ro');  
  lh = line(rpw(1,:),rpw(2,:));  
  hold off;
  
  % Draw sensor points
  for i=1:numsens
    xws = xwsc{i};
    figure(fh);
    hold on;  sh = scatter(xws(1,:),xws(2,:),'bo');  hold off;
  end

  % Draw sensor lines
  for i=1:numsens
    xw = xwc{i};
    figure(fh);
    hold on;  sh = scatter(xw(1,:),xw(2,:),'b.');  hold off;
  end

  % Draw collision points
  for i=1:numsens
    xwcoll = xwcollc{i};
    hold on;  sh = scatter(xwcoll(1),xwcoll(2),'gx');  hold off;
    set(sh,'SizeData',100,'LineWidth',2);
  end

  % Terminate simulation to prevent too many figure windows
  %modelName = get_param(bdroot, 'Name');
  %set_param(modelName,'SimulationCommand','stop');
  error('Terminating simulation to prevent too many figures');
end

== matlab function mmuct_lib/mm pwm to w ==
  data: pwm_R input; w_R output; pwm_L input; w_L output; deadb parameter; maxw parameter
function [w_R,w_L] = pwm2angfreq(pwm_R,pwm_L,deadb, maxw)

a = maxw/(100-deadb);
c = -deadb*maxw/(100-deadb);

% Piecewise (approximate)
if pwm_R<-deadb
  w_R = a*pwm_R - c;
elseif pwm_R<deadb
  w_R = 0;
else
  w_R = a*pwm_R + c;
end

% Piecewise (approximate)
if pwm_L<-deadb
  w_L = a*pwm_L - c;
elseif pwm_L<deadb
  w_L = 0;
else
  w_L = a*pwm_L + c;
end

== matlab function mmuct_lib/mm basic IMU/IMU acceleration ==
  data: As output; Ai output; Rsl output; Rlr input; A input; w input; alpha input; simstruct parameter
function [As,Ai,Rsl]  = getimuaccel(Rlr,A,w,alpha,simstruct)
%GETIMUACCEL  Get linear acceleration of IMU in local frame
%  [As,Ai,Rls]  = getimuaccel(Rlr,A,w,alpha,simstruct) calculates the linear
%  acceleration at the origin of an IMU sensor frame fixed to a robot.  The
%  robot frame is oriented by Rlr with respect to the local frame and is
%  moving according to (A,w,alpha) = (linear acceleration,angular
%  velocity,anglular acceleration). 
%
%  The function returns the linear acceleration As and the orientation Rsl
%  of the local frame in the sensor frame.  These two outputs are useful
%  for setting up the standard Simulink IMU block.

% Checks
if size(A,1)~=1 || size(A,2)~=3, error('Input A must be 1x3'); end
if size(w,1)~=1 || size(w,2)~=3, error('Input w must be 1x3'); end
if size(alpha,1)~=1 || size(alpha,2)~=3, error('Input alpha must be 1x3'); end

% Get sensor location vector (r_i-R) in local frame
si = Rlr*simstruct.timu;

% Kinematic equation (https://en.wikipedia.org/wiki/Rigid_body_dynamics,
% taking R as origin of robot frame).  This find the linear acceleration of
% the IMU in the local (inertial) navigation frame 
Ai = cross(alpha,si) + cross(w,cross(w,si)) + A;

% Get sensor orientation in local frame
Rrs = simstruct.Rimu;
Rls = Rlr*Rrs;
Rsl = inv(Rls);

% Generate measurements in sensor frame
Ait = Ai;  Ait(3) = Ait(3) + 9.81;  % add gravity
As = (inv(Rls)*Ait')';  
ws = (inv(Rls)*w')';
